simulink model "Guidance_ASMC"  (R2020a)
settings: Solver=ode1  StartTime=0.0  StopTime=50  FixedStep=0.001  RelTol=1e-3
libraries: simulink x1
settings Model: Creator=franc  LastModifiedBy=Sebas
settings SolverCC: ZeroCrossAlgorithm=Adaptive
settings DebuggingCC: IgnoredZcDiagnostic=none
settings ModelReferenceCC: ModelReferenceMinAlgLoopOccurrences=on

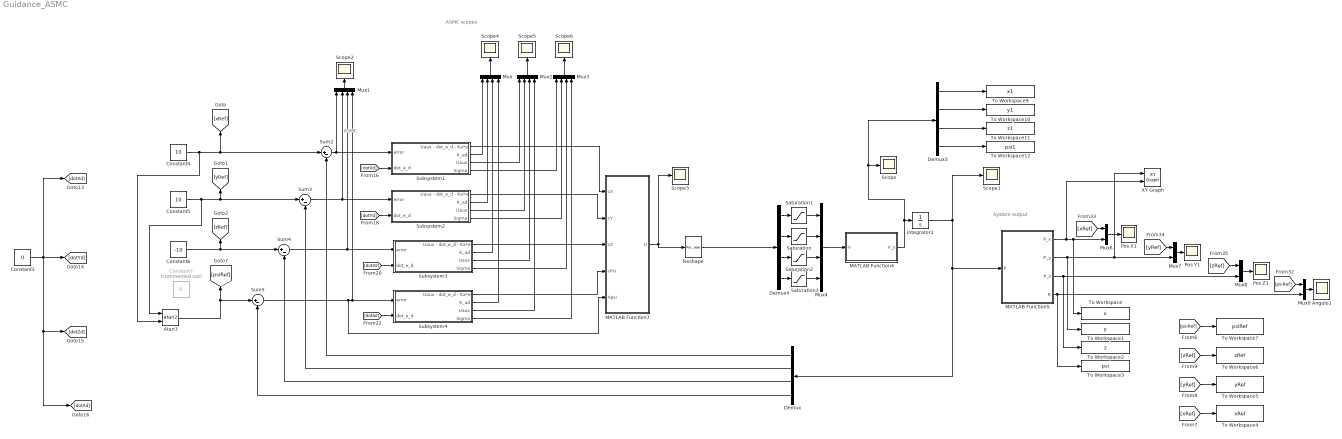
== system Guidance_ASMC ==
  note: ASMC scopes
  note: System output
  note: ASMC
  Angulo1 : Scope
  Atan3 : Trigonometry  Operator=atan2
  Constant3 : Constant  Value=0
  Constant4 : Constant  Value=10
  Constant5 : Constant  Value=10
  Constant6 : Constant  Value=-10
  Constant7 : Constant  Commented=on  Value=0
  Demux : Demux
  Demux3 : Demux
  Demux4 : Demux
  Integrator2 : Integrator
  MATLAB Function4 : MATLAB Function  TreatAsAtomicUnit=on
      settings: MinAlgLoopOccurrences=on
  MATLAB Function5 : MATLAB Function  TreatAsAtomicUnit=on
  MATLAB Function7 : MATLAB Function  TreatAsAtomicUnit=on
      settings: MinAlgLoopOccurrences=on
  Mux{,1..4} (5 alike) : Mux
  Mux{6..9} (4 alike) : Mux  Inputs=2
  Pos X1 : Scope
  Pos Y1 : Scope
  Pos Z1 : Scope
  Reshape : Reshape  OutputDimensionality=Customize  OutputDimensions=[4,1]
  Saturation : Saturate  UpperLimit=1.5  LowerLimit=-1.5
  Saturation1 : Saturate  UpperLimit=0.94  LowerLimit=-0.94
  Saturation2 : Saturate  UpperLimit=0.671  LowerLimit=-0.66
  Saturation3 : Saturate  UpperLimit=4.245  LowerLimit=-4.245
  Scope{,1..6} (7 alike) : Scope
  Subsystem1 : Subsystem  mask{Ka=0.001, K2=0.01, Beta=0.01, Mu=0.1, Kmin=0.01}
  Subsystem2 : Subsystem  mask{Ka=0.001, K2=0.01, Beta=0.01, Mu=0.1, Kmin=0.01}
  Subsystem3 : Subsystem  mask{Ka=0.001, K2=0.01, Beta=0.01, Mu=0.1, Kmin=0.01}
  Subsystem4 : Subsystem  mask{Ka=0.001, K2=0.01, Beta=0.1, Mu=0.1, Kmin=0.01}
  Sum{2..5} (4 alike) : Sum  Inputs=|+-
  To Workspace : ToWorkspace  VariableName=x  SampleTime=-1
      settings: Save2DSignal=2-D array (concatenate along first dimension)
  To Workspace1 : ToWorkspace  VariableName=y  SampleTime=-1
      settings: Save2DSignal=2-D array (concatenate along first dimension)
  To Workspace10 : ToWorkspace  VariableName=y1  SampleTime=-1
      settings: Save2DSignal=2-D array (concatenate along first dimension)
  To Workspace11 : ToWorkspace  VariableName=z1  SampleTime=-1
      settings: Save2DSignal=2-D array (concatenate along first dimension)
  To Workspace12 : ToWorkspace  VariableName=psi1  SampleTime=-1
      settings: Save2DSignal=2-D array (concatenate along first dimension)
  To Workspace2 : ToWorkspace  VariableName=z  SampleTime=-1
      settings: Save2DSignal=2-D array (concatenate along first dimension)
  To Workspace3 : ToWorkspace  VariableName=psi  SampleTime=-1
      settings: Save2DSignal=2-D array (concatenate along first dimension)
  To Workspace4 : ToWorkspace  VariableName=xRef  SampleTime=-1
      settings: Save2DSignal=2-D array (concatenate along first dimension)
  To Workspace5 : ToWorkspace  VariableName=yRef  SampleTime=-1
      settings: Save2DSignal=2-D array (concatenate along first dimension)
  To Workspace6 : ToWorkspace  VariableName=zRef  SampleTime=-1
      settings: Save2DSignal=2-D array (concatenate along first dimension)
  To Workspace7 : ToWorkspace  VariableName=psiRef  SampleTime=-1
      settings: Save2DSignal=2-D array (concatenate along first dimension)
  To Workspace9 : ToWorkspace  VariableName=x1  SampleTime=-1
      settings: Save2DSignal=2-D array (concatenate along first dimension)
  XY Graph : simulink/Sinks/XY Graph  xmin=-15  xmax=15  ymin=-15  ymax=15  st=-1
  wires:
  MATLAB Function5/1(P_x) -> XY Graph/2, Mux6/2, To Workspace/1
  MATLAB Function5/2(P_y) -> Mux7/2, XY Graph/1, To Workspace1/1
  MATLAB Function5/3(P_z) -> To Workspace2/1, Mux8/2
  MATLAB Function5/4(R) -> Mux9/2, To Workspace3/1
  Mux6/1 -> Pos X1/1
  Mux7/1 -> Pos Y1/1
  Mux8/1 -> Pos Z1/1
  Mux9/1 -> Angulo1/1
  [xRef] -> To Workspace4/1
  [yRef] -> To Workspace5/1
  [psiRef] -> To Workspace7/1
  [zRef] -> To Workspace6/1
  [xRef] -> Mux6/1
  [yRef] -> Mux7/1
  [zRef] -> Mux8/1
  [psiRef] -> Mux9/1
  Integrator2/1 -> Scope1/1, Demux/1, MATLAB Function5/1(P)
  Demux/1 -> Sum2/2
  Demux/2 -> Sum3/2
  MATLAB Function7/1(U) -> Reshape/1, Scope3/1
  [dotXd] -> Subsystem1/2(dot_e_d)
  Sum2/1 -> Subsystem1/1(error), Mux1/1
  Sum3/1 -> Subsystem2/1(error), Mux1/2
  Sum4/1 -> Subsystem3/1(error), Mux1/3
  [dotYd] -> Subsystem2/2(dot_e_d)
  [dotZd] -> Subsystem3/2(dot_e_d)
  [dotAd] -> Subsystem4/2(dot_e_d)
  Subsystem1/1(Uaux - dot_e_d - Ka*e) -> MATLAB Function7/1(cX)
  Subsystem2/1(Uaux - dot_e_d - Ka*e) -> MATLAB Function7/2(cY)
  Subsystem3/1(Uaux - dot_e_d - Ka*e) -> MATLAB Function7/3(cZ)
  Subsystem4/1(Uaux - dot_e_d - Ka*e) -> MATLAB Function7/4(cPsi)
  Demux/3 -> Sum4/2
  Demux/4 -> Sum5/2
  Sum5/1 -> Subsystem4/1(error), Mux1/4, MATLAB Function7/5(Apsi)
  Reshape/1 -> Demux4/1
  Demux3/2 -> To Workspace10/1
  Demux3/3 -> To Workspace11/1
  Demux3/4 -> To Workspace12/1
  Demux3/1 -> To Workspace9/1
  Subsystem1/2(K_ad) -> Mux/1
  Subsystem2/2(K_ad) -> Mux/2
  Subsystem3/2(K_ad) -> Mux/3
  Subsystem4/2(K_ad) -> Mux/4
  Subsystem1/3(Uaux) -> Mux2/1
  Subsystem2/3(Uaux) -> Mux2/2
  Subsystem3/3(Uaux) -> Mux2/3
  Subsystem4/3(Uaux) -> Mux2/4
  Subsystem1/4(Sigma) -> Mux3/1
  Subsystem2/4(Sigma) -> Mux3/2
  Subsystem3/4(Sigma) -> Mux3/3
  Subsystem4/4(Sigma) -> Mux3/4
  Mux/1 -> Scope4/1
  Mux2/1 -> Scope5/1
  Mux3/1 -> Scope6/1
  Constant3/1 -> [dotAd], [dotZd], [dotXd], [dotYd]
  Constant4/1 -> Atan3/2, [xRef], Sum2/1
  Constant5/1 -> Atan3/1, Sum3/1, [yRef]
  Constant6/1 -> Sum4/1, [zRef]
  MATLAB Function4/1(V_s) -> Demux3/1, Scope/1, Integrator2/1
  Demux4/1 -> Saturation1/1
  Saturation3/1 -> Mux4/4
  Demux4/3 -> Saturation2/1
  Saturation2/1 -> Mux4/3
  Demux4/2 -> Saturation/1
  Saturation/1 -> Mux4/2
  Saturation1/1 -> Mux4/1
  Demux4/4 -> Saturation3/1
  Mux4/1 -> MATLAB Function4/1(V)
  Mux1/1 -> Scope2/1
  Atan3/1 -> Sum5/1, [psiRef]

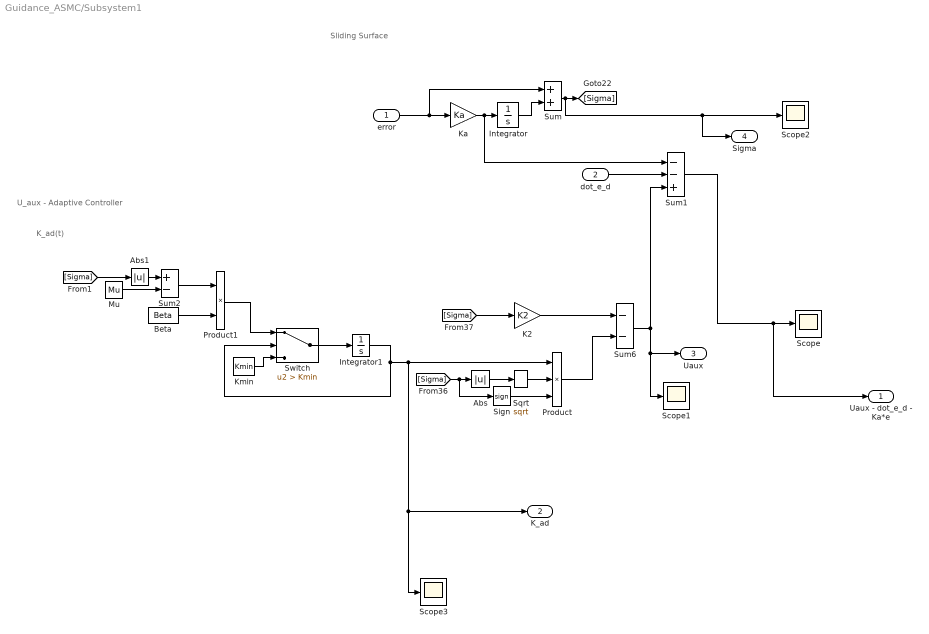
== system Guidance_ASMC/Subsystem1 ==
  note: K_ad(t)
  note: Sliding Surface
  note: U_aux - Adaptive Controller
  error : Inport
  dot_e_d : Inport  Port=2
  Abs : Abs
  Abs1 : Abs
  Beta : Constant  Value=Beta
  Integrator : Integrator
  Integrator1 : Integrator
  K2 : Gain  Gain=K2
  Ka : Gain  Gain=Ka
  Kmin : Constant  Value=Kmin
  Mu : Constant  Value=Mu
  Product : Product  Inputs=3
  Product1 : Product
  Scope{,1..3} (4 alike) : Scope
  Sign : Signum
  Sqrt : Sqrt  SaturateOnIntegerOverflow=on
  Sum : Sum
  Sum1 : Sum  Inputs=--+
  Sum2 : Sum  Inputs=+-
  Sum6 : Sum  Inputs=--
  Switch : Switch  Criteria=u2 > Threshold  Threshold=Kmin
  Uaux - dot_e_d - Ka*e : Outport
  K_ad : Outport  Port=2
  Uaux : Outport  Port=3
  Sigma : Outport  Port=4
  wires:
  Product1/1 -> Switch/1
  Sum2/1 -> Product1/1
  Beta/1 -> Product1/2
  Mu/1 -> Sum2/2
  Abs1/1 -> Sum2/1
  [Sigma] -> Abs1/1
  Kmin/1 -> Switch/3
  Integrator1/1 -> Switch/2, Product/1, K_ad/1, Scope3/1
  Switch/1 -> Integrator1/1
  dot_e_d/1 -> Sum1/2
  Sum1/1 -> Scope/1, Uaux - dot_e_d - Ka*e/1
  Sqrt/1 -> Product/2
  Sign/1 -> Product/3
  Sum/1 -> [Sigma], Scope2/1, Sigma/1
  K2/1 -> Sum6/1
  Abs/1 -> Sqrt/1
  Product/1 -> Sum6/2
  [Sigma] -> Abs/1, Sign/1
  Sum6/1 -> Sum1/3, Uaux/1, Scope1/1
  Ka/1 -> Integrator/1, Sum1/1
  [Sigma] -> K2/1
  error/1 -> Ka/1, Sum/1
  Integrator/1 -> Sum/2

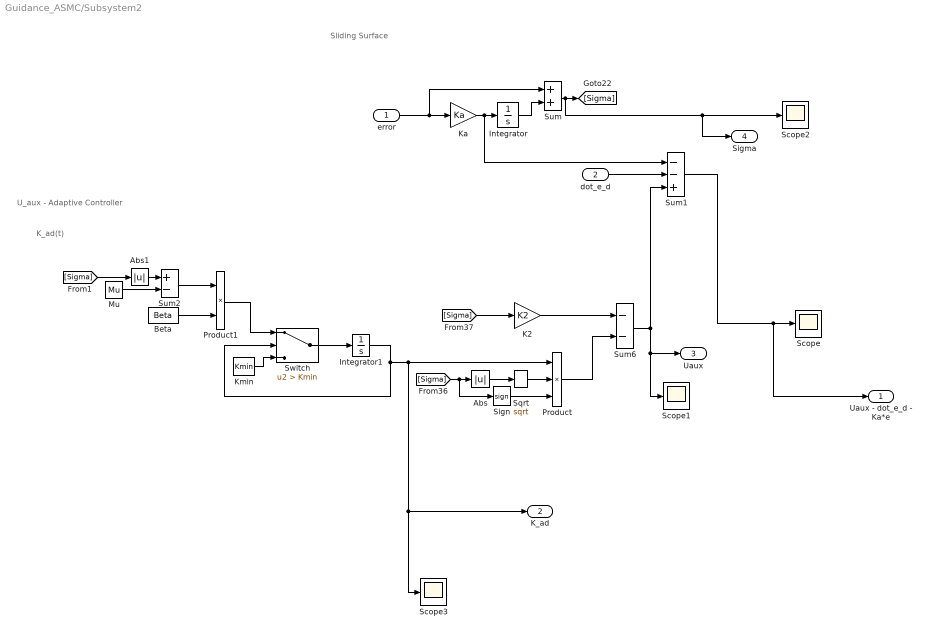
== system Guidance_ASMC/Subsystem2 ==
  note: U_aux - Adaptive Controller
  note: Sliding Surface
  note: K_ad(t)
  error : Inport
  dot_e_d : Inport  Port=2
  Abs : Abs
  Abs1 : Abs
  Beta : Constant  Value=Beta
  Integrator : Integrator
  Integrator1 : Integrator
  K2 : Gain  Gain=K2
  Ka : Gain  Gain=Ka
  Kmin : Constant  Value=Kmin
  Mu : Constant  Value=Mu
  Product : Product  Inputs=3
  Product1 : Product
  Scope{,1..3} (4 alike) : Scope
  Sign : Signum
  Sqrt : Sqrt  SaturateOnIntegerOverflow=on
  Sum : Sum
  Sum1 : Sum  Inputs=--+
  Sum2 : Sum  Inputs=+-
  Sum6 : Sum  Inputs=--
  Switch : Switch  Criteria=u2 > Threshold  Threshold=Kmin
  Uaux - dot_e_d - Ka*e : Outport
  K_ad : Outport  Port=2
  Uaux : Outport  Port=3
  Sigma : Outport  Port=4
  wires:
  Integrator/1 -> Sum/2
  error/1 -> Sum/1, Ka/1
  [Sigma] -> K2/1
  Ka/1 -> Sum1/1, Integrator/1
  Sum6/1 -> Scope1/1, Uaux/1, Sum1/3
  [Sigma] -> Sign/1, Abs/1
  Product/1 -> Sum6/2
  Abs/1 -> Sqrt/1
  K2/1 -> Sum6/1
  Sum/1 -> Sigma/1, Scope2/1, [Sigma]
  Sign/1 -> Product/3
  Sqrt/1 -> Product/2
  Sum1/1 -> Uaux - dot_e_d - Ka*e/1, Scope/1
  dot_e_d/1 -> Sum1/2
  Switch/1 -> Integrator1/1
  Integrator1/1 -> Scope3/1, K_ad/1, Product/1, Switch/2
  Kmin/1 -> Switch/3
  [Sigma] -> Abs1/1
  Abs1/1 -> Sum2/1
  Mu/1 -> Sum2/2
  Beta/1 -> Product1/2
  Sum2/1 -> Product1/1
  Product1/1 -> Switch/1

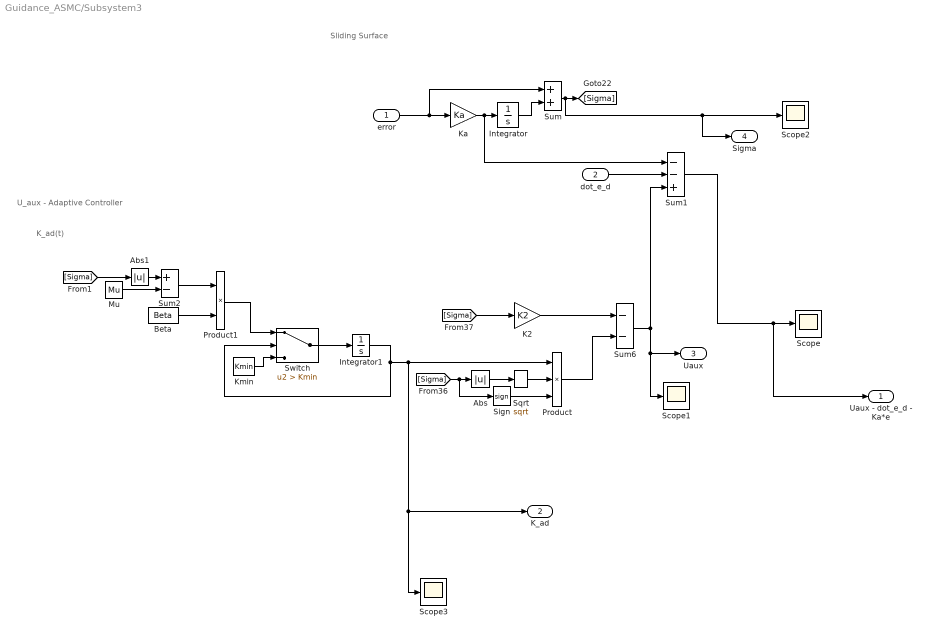
== system Guidance_ASMC/Subsystem3 ==
  note: K_ad(t)
  note: Sliding Surface
  note: U_aux - Adaptive Controller
  error : Inport
  dot_e_d : Inport  Port=2
  Abs : Abs
  Abs1 : Abs
  Beta : Constant  Value=Beta
  Integrator : Integrator
  Integrator1 : Integrator
  K2 : Gain  Gain=K2
  Ka : Gain  Gain=Ka
  Kmin : Constant  Value=Kmin
  Mu : Constant  Value=Mu
  Product : Product  Inputs=3
  Product1 : Product
  Scope{,1..3} (4 alike) : Scope
  Sign : Signum
  Sqrt : Sqrt  SaturateOnIntegerOverflow=on
  Sum : Sum
  Sum1 : Sum  Inputs=--+
  Sum2 : Sum  Inputs=+-
  Sum6 : Sum  Inputs=--
  Switch : Switch  Criteria=u2 > Threshold  Threshold=Kmin
  Uaux - dot_e_d - Ka*e : Outport
  K_ad : Outport  Port=2
  Uaux : Outport  Port=3
  Sigma : Outport  Port=4
  wires:
  Product1/1 -> Switch/1
  Sum2/1 -> Product1/1
  Beta/1 -> Product1/2
  Mu/1 -> Sum2/2
  Abs1/1 -> Sum2/1
  [Sigma] -> Abs1/1
  Kmin/1 -> Switch/3
  Integrator1/1 -> Switch/2, Product/1, K_ad/1, Scope3/1
  Switch/1 -> Integrator1/1
  dot_e_d/1 -> Sum1/2
  Sum1/1 -> Scope/1, Uaux - dot_e_d - Ka*e/1
  Sqrt/1 -> Product/2
  Sign/1 -> Product/3
  Sum/1 -> [Sigma], Scope2/1, Sigma/1
  K2/1 -> Sum6/1
  Abs/1 -> Sqrt/1
  Product/1 -> Sum6/2
  [Sigma] -> Abs/1, Sign/1
  Sum6/1 -> Sum1/3, Uaux/1, Scope1/1
  Ka/1 -> Integrator/1, Sum1/1
  [Sigma] -> K2/1
  error/1 -> Ka/1, Sum/1
  Integrator/1 -> Sum/2

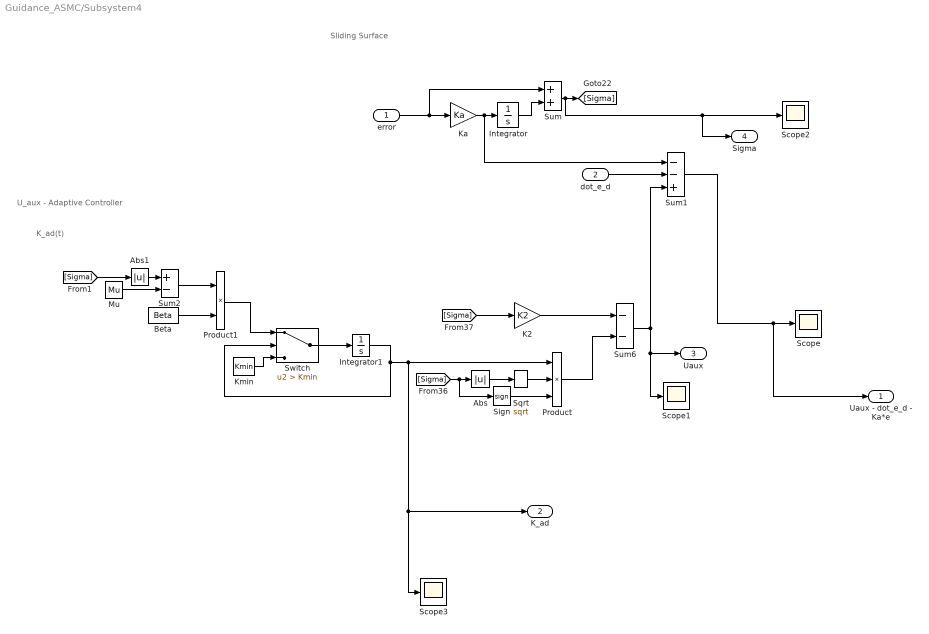
== system Guidance_ASMC/Subsystem4 ==
  note: U_aux - Adaptive Controller
  note: Sliding Surface
  note: K_ad(t)
  error : Inport
  dot_e_d : Inport  Port=2
  Abs : Abs
  Abs1 : Abs
  Beta : Constant  Value=Beta
  Integrator : Integrator
  Integrator1 : Integrator
  K2 : Gain  Gain=K2
  Ka : Gain  Gain=Ka
  Kmin : Constant  Value=Kmin
  Mu : Constant  Value=Mu
  Product : Product  Inputs=3
  Product1 : Product
  Scope{,1..3} (4 alike) : Scope
  Sign : Signum
  Sqrt : Sqrt  SaturateOnIntegerOverflow=on
  Sum : Sum
  Sum1 : Sum  Inputs=--+
  Sum2 : Sum  Inputs=+-
  Sum6 : Sum  Inputs=--
  Switch : Switch  Criteria=u2 > Threshold  Threshold=Kmin
  Uaux - dot_e_d - Ka*e : Outport
  K_ad : Outport  Port=2
  Uaux : Outport  Port=3
  Sigma : Outport  Port=4
  wires:
  Integrator/1 -> Sum/2
  error/1 -> Sum/1, Ka/1
  [Sigma] -> K2/1
  Ka/1 -> Sum1/1, Integrator/1
  Sum6/1 -> Scope1/1, Uaux/1, Sum1/3
  [Sigma] -> Sign/1, Abs/1
  Product/1 -> Sum6/2
  Abs/1 -> Sqrt/1
  K2/1 -> Sum6/1
  Sum/1 -> Sigma/1, Scope2/1, [Sigma]
  Sign/1 -> Product/3
  Sqrt/1 -> Product/2
  Sum1/1 -> Uaux - dot_e_d - Ka*e/1, Scope/1
  dot_e_d/1 -> Sum1/2
  Switch/1 -> Integrator1/1
  Integrator1/1 -> Scope3/1, K_ad/1, Product/1, Switch/2
  Kmin/1 -> Switch/3
  [Sigma] -> Abs1/1
  Abs1/1 -> Sum2/1
  Mu/1 -> Sum2/2
  Beta/1 -> Product1/2
  Sum2/1 -> Product1/1
  Product1/1 -> Switch/1

== matlab function Guidance_ASMC/MATLAB Function4 ==
  data: V input; V_s output
function V_s = Modelo(V)
dotx = V(1,1)*cos(V(4,1)) - V(2,1)*sin(V(4,1));
doty = V(1,1)*sin(V(4,1)) + V(2,1)*cos(V(4,1));
dotz = V(3,1);
W = V(4,1);
V_s = [dotx,doty,dotz,W];

== matlab function Guidance_ASMC/MATLAB Function5 ==
  data: P input; P_x output; P_y output; P_z output; R output
function [P_x,P_y,P_z,R] = Posicion(P)
P_x=P(1,1);
P_y=P(1,2);
P_z=P(1,3);
R=P(1,4);

== matlab function Guidance_ASMC/MATLAB Function7 ==
  data: cX input; U output; cY input; cZ input; cPsi input; Apsi input
function U = G(cX,cY,cZ,cPsi,Apsi)
Aux = [cos(Apsi), sin(Apsi), 0, 0;
       -sin(Apsi), cos(Apsi), 0 , 0;
       0 , 0 , 1 , 0;
       0 , 0 , 0 , 1];
C = [cX,cY,cZ,cPsi]'; 
U = -1*Aux*C;
